simulink library "AMK_comms_plant_lib"  (R2022b)
settings: Solver=VariableStepAuto  StartTime=0.0  StopTime=10.0  RelTol=1e-3
libraries: dspstat3 x4, simulink x2
settings Model: Creator=LinF  LastModifiedBy=LinF

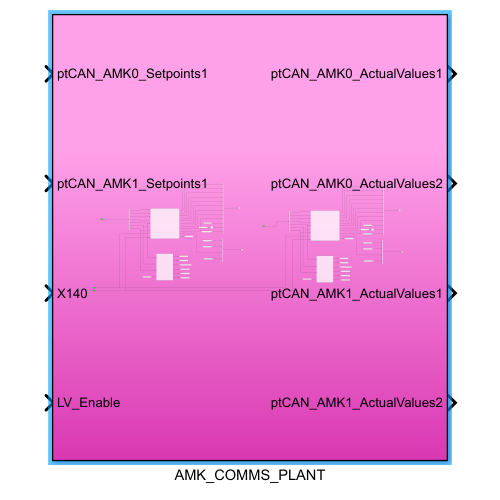
[thumbnail: Simulink's stored preview of the top-level diagram]
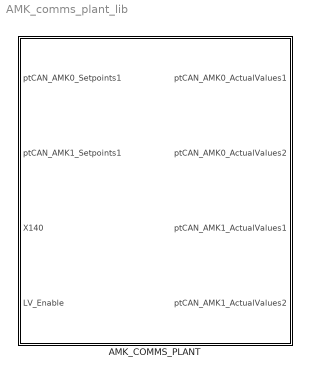
== system AMK_comms_plant_lib ==
  AMK_COMMS_PLANT : Subsystem

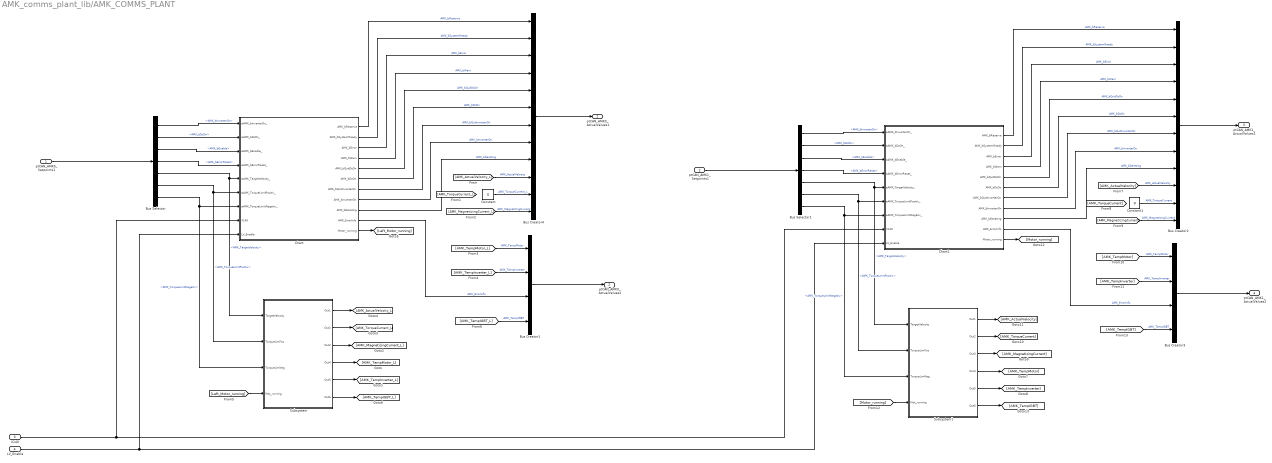
== system AMK_comms_plant_lib/AMK_COMMS_PLANT ==
  ptCAN_AMK0_Setpoints1 : Inport
  ptCAN_AMK1_Setpoints1 : Inport  Port=2
  X140 : Inport  Port=3
  LV_Enable : Inport  Port=4
  Bus Creator1 : BusCreator  Inputs=4
  Bus Creator2 : BusCreator  Inputs=12
  Bus Creator3 : BusCreator  Inputs=4
  Bus Creator4 : BusCreator  Inputs=12
  Bus Selector : BusSelector  OutputSignals=AMK_bInverterOn,AMK_bDcOn,AMK_bEnable,AMK_bErrorReset,AMK_TargetVelocity,AMK_TorqueLimitPositiv,AMK_TorqueLimitNegativ
  Bus Selector1 : BusSelector  OutputSignals=AMK_bInverterOn,AMK_bDcOn,AMK_bEnable,AMK_bErrorReset,AMK_TargetVelocity,AMK_TorqueLimitPositiv,AMK_TorqueLimitNegativ
  Chart : Stateflow chart  TreatAsAtomicUnit=on
  Chart1 : Stateflow chart  TreatAsAtomicUnit=on
  Constant : Constant  Value=0
  Constant1 : Constant  Value=0
  Subsystem : Subsystem
  Subsystem1 : Subsystem
  ptCAN_AMK0_ActualValues1 : Outport
  ptCAN_AMK0_ActualValues2 : Outport  Port=2
  ptCAN_AMK1_ActualValues1 : Outport  Port=3
  ptCAN_AMK1_ActualValues2 : Outport  Port=4
  wires:
  Subsystem/6(Out6) -> [AMK_TempIGBT_L]
  Subsystem/1(Out1) -> [AMK_ActualVelocity_L]
  Subsystem/2(Out2) -> [AMK_TorqueCurrent_L]
  Subsystem/3(Out3) -> [AMK_MagnetizingCurrent_L]
  Subsystem/4(Out4) -> [AMK_TempMotor_L]
  Subsystem/5(Out5) -> [AMK_TempInverter_L]
  [Left_Motor_running] -> Subsystem/4(Mot_running)
  Chart/11(Motor_running) -> [Left_Motor_running]
  Bus Selector/7 -> Subsystem/3(TorqueLimNeg), Chart/7(aAMK_TorqueLimitNegativ_)  "<AMK_TorqueLimitNegativ>"
  Bus Selector/6 -> Subsystem/2(TorqueLimPos), Chart/6(aAMK_TorqueLimitPositiv_)  "<AMK_TorqueLimitPositiv>"
  Bus Selector/5 -> Subsystem/1(TargetVelocity), Chart/5(aAMK_TargetVelocity_)  "<AMK_TargetVelocity>"
  Bus Selector/4 -> Chart/4(aAMK_bErrorReset_)  "<AMK_bErrorReset>"
  Bus Selector/3 -> Chart/3(aAMK_bEnable_)  "<AMK_bEnable>"
  Bus Selector/2 -> Chart/2(aAMK_bDcOn_)  "<AMK_bDcOn>"
  Bus Selector/1 -> Chart/1(aAMK_bInverterOn_)  "<AMK_bInverterOn>"
  ptCAN_AMK0_Setpoints1/1 -> Bus Selector/1
  Bus Creator1/1 -> ptCAN_AMK0_ActualValues2/1
  [AMK_TempMotor_L] -> Bus Creator1/1  "AMK_TempMotor"
  [AMK_TempIGBT_L] -> Bus Creator1/4  "AMK_TempIGBT"
  [AMK_TempInverter_L] -> Bus Creator1/2  "AMK_TempInverter"
  Chart/10(AMK_ErrorInfo) -> Bus Creator1/3  "AMK_ErrorInfo"
  LV_Enable/1 -> Chart1/9(LV_Enable), Chart/9(LV_Enable)
  Chart1/7(AMK_bQuitInverterOn) -> Bus Creator2/7  "AMK_bQuitInverterOn"
  [Motor_running] -> Subsystem1/4(Mot_running)
  X140/1 -> Chart/8(X140), Chart1/8(X140)
  Chart1/4(AMK_bWarn) -> Bus Creator2/4  "AMK_bWarn"
  Bus Creator2/1 -> ptCAN_AMK1_ActualValues1/1
  Chart1/10(AMK_ErrorInfo) -> Bus Creator3/3  "AMK_ErrorInfo"
  Chart1/6(AMK_bDcOn) -> Bus Creator2/6  "AMK_bDcOn"
  Chart1/1(AMK_bReserve) -> Bus Creator2/1  "AMK_bReserve"
  [AMK_TempInverter] -> Bus Creator3/2  "AMK_TempInverter"
  Bus Selector1/7 -> Subsystem1/3(TorqueLimNeg), Chart1/7(aAMK_TorqueLimitNegativ_)  "<AMK_TorqueLimitNegativ>"
  Chart1/3(AMK_bError) -> Bus Creator2/3  "AMK_bError"
  Chart1/9(AMK_bDerating) -> Bus Creator2/9  "AMK_bDerating"
  ptCAN_AMK1_Setpoints1/1 -> Bus Selector1/1
  Bus Selector1/4 -> Chart1/4(aAMK_bErrorReset_)  "<AMK_bErrorReset>"
  Bus Selector1/2 -> Chart1/2(aAMK_bDcOn_)  "<AMK_bDcOn>"
  [AMK_TempIGBT] -> Bus Creator3/4  "AMK_TempIGBT"
  Chart1/5(AMK_bQuitDcOn) -> Bus Creator2/5  "AMK_bQuitDcOn"
  Bus Selector1/1 -> Chart1/1(aAMK_bInverterOn_)  "<AMK_bInverterOn>"
  Subsystem1/3(Out3) -> [AMK_MagnetizingCurrent]
  Chart1/2(AMK_bSystemReady) -> Bus Creator2/2  "AMK_bSystemReady"
  Bus Selector1/5 -> Subsystem1/1(TargetVelocity), Chart1/5(aAMK_TargetVelocity_)  "<AMK_TargetVelocity>"
  [AMK_TempMotor] -> Bus Creator3/1  "AMK_TempMotor"
  Subsystem1/1(Out1) -> [AMK_ActualVelocity]
  Chart1/8(AMK_bInverterOn) -> Bus Creator2/8  "AMK_bInverterOn"
  Subsystem1/2(Out2) -> [AMK_TorqueCurrent]
  Subsystem1/6(Out6) -> [AMK_TempIGBT]
  Bus Selector1/3 -> Chart1/3(aAMK_bEnable_)  "<AMK_bEnable>"
  Subsystem1/5(Out5) -> [AMK_TempInverter]
  Chart1/11(Motor_running) -> [Motor_running]
  [AMK_ActualVelocity] -> Bus Creator2/10  "AMK_ActualVelocity"
  Subsystem1/4(Out4) -> [AMK_TempMotor]
  Bus Selector1/6 -> Subsystem1/2(TorqueLimPos), Chart1/6(aAMK_TorqueLimitPositiv_)  "<AMK_TorqueLimitPositiv>"
  Bus Creator3/1 -> ptCAN_AMK1_ActualValues2/1
  [AMK_MagnetizingCurrent] -> Bus Creator2/12  "AMK_MagnetizingCurrent"
  Chart/7(AMK_bQuitInverterOn) -> Bus Creator4/7  "AMK_bQuitInverterOn"
  [AMK_ActualVelocity_L] -> Bus Creator4/10  "AMK_ActualVelocity"
  Chart/8(AMK_bInverterOn) -> Bus Creator4/8  "AMK_bInverterOn"
  Chart/5(AMK_bQuitDcOn) -> Bus Creator4/5  "AMK_bQuitDcOn"
  Chart/2(AMK_bSystemReady) -> Bus Creator4/2  "AMK_bSystemReady"
  Chart/4(AMK_bWarn) -> Bus Creator4/4  "AMK_bWarn"
  Chart/9(AMK_bDerating) -> Bus Creator4/9  "AMK_bDerating"
  Chart/6(AMK_bDcOn) -> Bus Creator4/6  "AMK_bDcOn"
  Chart/3(AMK_bError) -> Bus Creator4/3  "AMK_bError"
  Bus Creator4/1 -> ptCAN_AMK0_ActualValues1/1
  [AMK_MagnetizingCurrent_L] -> Bus Creator4/12  "AMK_MagnetizingCurrent"
  Chart/1(AMK_bReserve) -> Bus Creator4/1  "AMK_bReserve"
  Constant/1 -> Bus Creator4/11  "AMK_TorqueCurrent_L"
  Constant1/1 -> Bus Creator2/11  "AMK_TorqueCurrent"

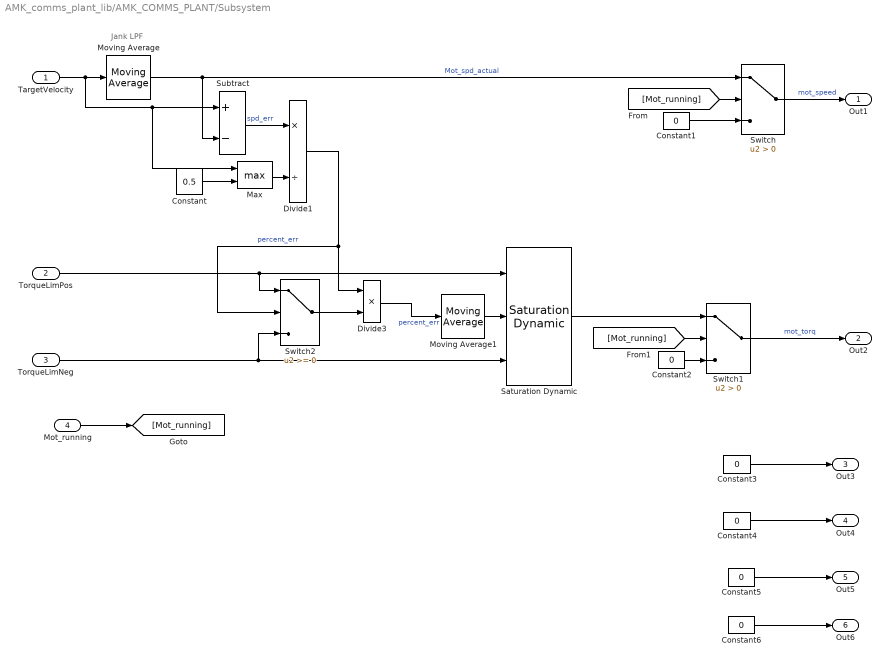
== system AMK_comms_plant_lib/AMK_COMMS_PLANT/Subsystem ==
  note: Jank LPF
  TargetVelocity : Inport
  TorqueLimPos : Inport  Port=2
  TorqueLimNeg : Inport  Port=3
  Mot_running : Inport  Port=4
  Constant : Constant  Value=0.5
  Constant1 : Constant  Value=0
  Constant2 : Constant  Value=0
  Constant{3..6} (4 alike) : Constant  Value=0  OutDataTypeStr=single
  Divide1 : Product  Inputs=*/
  Divide3 : Product  Inputs=**
  Max : MinMax  Function=max  Inputs=2
  Moving Average : dspstat3/Moving Average  Method=Sliding window  ForgettingFactorPort=off  SpecifyWindowLength=on  WindowLength=10  OverlapLength=9  AllowArbitraryInputLength=off  ForgettingFactor=0.9  SimulateUsing=Code generation
  Moving Average1 : dspstat3/Moving Average  Method=Sliding window  ForgettingFactorPort=off  SpecifyWindowLength=on  WindowLength=3  OverlapLength=2  AllowArbitraryInputLength=off  ForgettingFactor=0.9  SimulateUsing=Code generation
  Saturation Dynamic : simulink/Discontinuities/Saturation Dynamic  OutMin=[]  OutMax=[]  OutDataTypeStr=Inherit: Same as second input  OutDataType=fixdt(1, 16)  OutScaling=2^-10  DoSatur=off
  Subtract : Sum  Inputs=+-
  Switch : Switch  Criteria=u2 > Threshold  OutDataTypeStr=single  SaturateOnIntegerOverflow=off  InputSameDT=off
  Switch1 : Switch  Criteria=u2 > Threshold  OutDataTypeStr=single  SaturateOnIntegerOverflow=off  InputSameDT=off
  Switch2 : Switch  SaturateOnIntegerOverflow=off  InputSameDT=off
  Out1 : Outport
  Out2 : Outport  Port=2
  Out3 : Outport  Port=3
  Out4 : Outport  Port=4
  Out5 : Outport  Port=5
  Out6 : Outport  Port=6
  wires:
  Max/1 -> Divide1/2
  Constant/1 -> Max/2
  Constant6/1 -> Out6/1
  Divide3/1 -> Moving Average1/1  "percent_err"
  Moving Average1/1 -> Saturation Dynamic/2
  TorqueLimNeg/1 -> Saturation Dynamic/3, Switch2/3
  Switch2/1 -> Divide3/2
  TorqueLimPos/1 -> Switch2/1, Saturation Dynamic/1
  Constant5/1 -> Out5/1
  Constant4/1 -> Out4/1
  Constant3/1 -> Out3/1
  Divide1/1 -> Switch2/2, Divide3/1  "percent_err"
  TargetVelocity/1 -> Moving Average/1, Subtract/1, Max/1
  Subtract/1 -> Divide1/1  "spd_err"
  Switch1/1 -> Out2/1  "mot_torq"
  Saturation Dynamic/1 -> Switch1/1
  [Mot_running] -> Switch1/2
  Constant2/1 -> Switch1/3
  Moving Average/1 -> Subtract/2, Switch/1  "Mot_spd_actual"
  Constant1/1 -> Switch/3
  Switch/1 -> Out1/1  "mot_speed"
  [Mot_running] -> Switch/2
  Mot_running/1 -> [Mot_running]

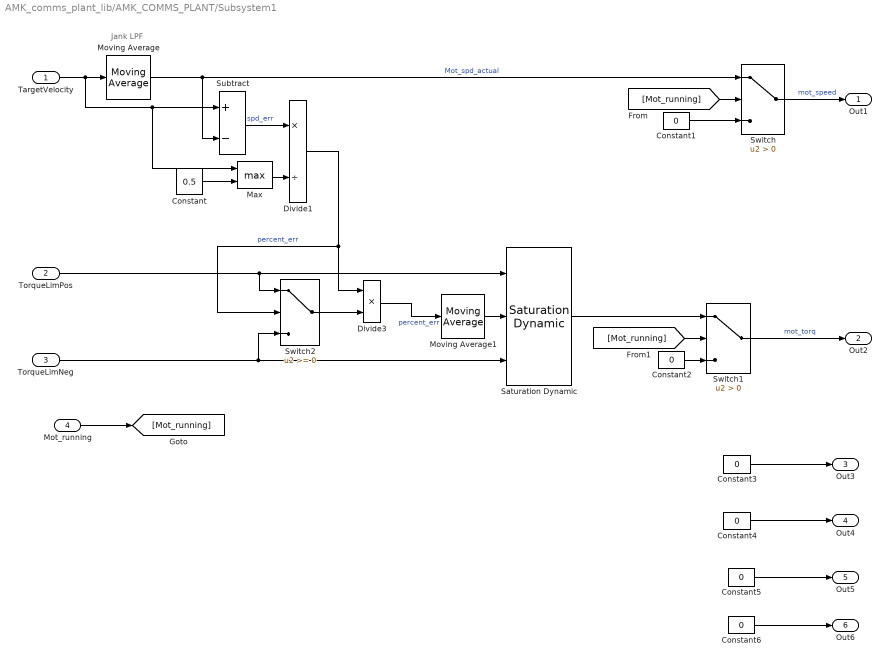
== system AMK_comms_plant_lib/AMK_COMMS_PLANT/Subsystem1 ==
  note: Jank LPF
  TargetVelocity : Inport
  TorqueLimPos : Inport  Port=2
  TorqueLimNeg : Inport  Port=3
  Mot_running : Inport  Port=4
  Constant : Constant  Value=0.5
  Constant1 : Constant  Value=0
  Constant2 : Constant  Value=0
  Constant{3..6} (4 alike) : Constant  Value=0  OutDataTypeStr=single
  Divide1 : Product  Inputs=*/
  Divide3 : Product  Inputs=**
  Max : MinMax  Function=max  Inputs=2
  Moving Average : dspstat3/Moving Average  Method=Sliding window  ForgettingFactorPort=off  SpecifyWindowLength=on  WindowLength=10  OverlapLength=9  AllowArbitraryInputLength=off  ForgettingFactor=0.9  SimulateUsing=Code generation
  Moving Average1 : dspstat3/Moving Average  Method=Sliding window  ForgettingFactorPort=off  SpecifyWindowLength=on  WindowLength=3  OverlapLength=2  AllowArbitraryInputLength=off  ForgettingFactor=0.9  SimulateUsing=Code generation
  Saturation Dynamic : simulink/Discontinuities/Saturation Dynamic  OutMin=[]  OutMax=[]  OutDataTypeStr=Inherit: Same as second input  OutDataType=fixdt(1, 16)  OutScaling=2^-10  DoSatur=off
  Subtract : Sum  Inputs=+-
  Switch : Switch  Criteria=u2 > Threshold  OutDataTypeStr=single  SaturateOnIntegerOverflow=off  InputSameDT=off
  Switch1 : Switch  Criteria=u2 > Threshold  OutDataTypeStr=single  SaturateOnIntegerOverflow=off  InputSameDT=off
  Switch2 : Switch  SaturateOnIntegerOverflow=off  InputSameDT=off
  Out1 : Outport
  Out2 : Outport  Port=2
  Out3 : Outport  Port=3
  Out4 : Outport  Port=4
  Out5 : Outport  Port=5
  Out6 : Outport  Port=6
  wires:
  Max/1 -> Divide1/2
  Constant/1 -> Max/2
  Constant6/1 -> Out6/1
  Divide3/1 -> Moving Average1/1  "percent_err"
  Moving Average1/1 -> Saturation Dynamic/2
  TorqueLimNeg/1 -> Saturation Dynamic/3, Switch2/3
  Switch2/1 -> Divide3/2
  TorqueLimPos/1 -> Switch2/1, Saturation Dynamic/1
  Constant5/1 -> Out5/1
  Constant4/1 -> Out4/1
  Constant3/1 -> Out3/1
  Divide1/1 -> Switch2/2, Divide3/1  "percent_err"
  TargetVelocity/1 -> Moving Average/1, Subtract/1, Max/1
  Subtract/1 -> Divide1/1  "spd_err"
  Switch1/1 -> Out2/1  "mot_torq"
  Saturation Dynamic/1 -> Switch1/1
  [Mot_running] -> Switch1/2
  Constant2/1 -> Switch1/3
  Moving Average/1 -> Subtract/2, Switch/1  "Mot_spd_actual"
  Constant1/1 -> Switch/3
  Switch/1 -> Out1/1  "mot_speed"
  [Mot_running] -> Switch/2
  Mot_running/1 -> [Mot_running]

== stateflow chart AMK_comms_plant_lib/AMK_COMMS_PLANT/Chart1 ==
  state AMK_idle
    en:
    AMK_bReserve = 0;
    AMK_bSystemReady = 0;
    AMK_bError = 0;
    AMK_bWarn = 0;
    AMK_bQuitDcOn = 0;
    AMK_bDcOn = 0;
    AMK_bQuitInverterOn = 0;
    AMK_bInverterOn = 0;
    AMK_bDerating = 0;
    AMK_ErrorInfo = 0;
    Motor_running = false;
  state LV_ON
    state Enable_System_Ready
      en:
      AMK_bSystemReady = 1;
    state bQuitDcOff
      en:
      AMK_bQuitDcOn = 0
    state Enable_Quit_Dc_On
      en:
      AMK_bQuitDcOn = 1;
      AMK_bDcOn = 1;
    state bDcOff
      en:
      AMK_bDcOn = 0
    state Inverter_Stuff2
      % (*3) and %(*4)
    state Inverter
    state bEnable_off
      en:
      AMK_bQuitDcOn = 0
    state Inventer_On
      en:
      AMK_bInverterOn = 1;
    state bInverter_off
      en:
      AMK_bInverterOn = 0
    state Quit_Inventer_On
      en:
      AMK_bQuitInverterOn =1;
    state Motor_running
      en:
      Motor_running = true;
    state Shut_off_start
      en:
      AMK_bQuitInverterOn =0;
    (default) -> Enable_System_Ready
    Enable_System_Ready -> (junction 99) : [aAMK_bDcOn_ == 1]
    (junction 99) -> Enable_Quit_Dc_On : after(250,msec)
    bDcOff -> bQuitDcOff
    Enable_Quit_Dc_On -> Inverter : [(abs(aAMK_TargetVelocity_) == 0) && ...
        | (abs(aAMK_TorqueLimitPositiv_) == 0) && ...
        | (abs(aAMK_TorqueLimitNegativ_) == 0)]
    Inverter_Stuff2 -> bDcOff : [aAMK_bDcOn_ == 0]
    bEnable_off -> Inverter_Stuff2
    Inverter -> (junction 101) : [(aAMK_bEnable_ == 1) && ...
        | (aAMK_bInverterOn_ == 1)]
    (junction 101) -> Inventer_On : after(250,msec)
    bInverter_off -> bEnable_off : [aAMK_bEnable_ == 0]
    Inventer_On -> Quit_Inventer_On : [X140 == 1]
    Shut_off_start -> bInverter_off [order 2] : [aAMK_bInverterOn_ == 0]
    Shut_off_start -> Quit_Inventer_On [order 1] : [X140 == 1]
    Quit_Inventer_On -> Motor_running : after(250,msec)
    Motor_running -> Shut_off_start : [X140 == 0]
  (default) -> AMK_idle
  AMK_idle -> LV_ON : [LV_Enable == 1]
  LV_ON -> AMK_idle : [LV_Enable == 0]
  data: aAMK_bInverterOn_ input; aAMK_bDcOn_ input; aAMK_bEnable_ input; aAMK_bErrorReset_ input; aAMK_TargetVelocity_ input; aAMK_TorqueLimitPositiv_ input; aAMK_TorqueLimitNegativ_ input; AMK_bReserve output uint8; AMK_bSystemReady output uint8; AMK_bError output uint8; AMK_bWarn output uint8; AMK_bQuitDcOn output uint8; AMK_bDcOn output uint8; AMK_bQuitInverterOn output uint8; AMK_bInverterOn output uint8; AMK_bDerating output uint8; AMK_ErrorInfo output int32; Motor_running output boolean =false; X140 input; LV_Enable input

== stateflow chart AMK_comms_plant_lib/AMK_COMMS_PLANT/Chart ==
  state AMK_idle
    en:
    AMK_bReserve = 0;
    AMK_bSystemReady = 0;
    AMK_bError = 0;
    AMK_bWarn = 0;
    AMK_bQuitDcOn = 0;
    AMK_bDcOn = 0;
    AMK_bQuitInverterOn = 0;
    AMK_bInverterOn = 0;
    AMK_bDerating = 0;
    AMK_ErrorInfo = 0;
    Motor_running = false;
  state LV_ON
    state Enable_System_Ready
      en:
      AMK_bSystemReady = 1;
    state bQuitDcOff
      en:
      AMK_bQuitDcOn = 0
    state Enable_Quit_Dc_On
      en:
      AMK_bQuitDcOn = 1;
      AMK_bDcOn = 1;
    state bDcOff
      en:
      AMK_bDcOn = 0
    state Inverter_Stuff2
      % (*3) and %(*4)
    state Inverter
    state bEnable_off
      en:
      AMK_bQuitDcOn = 0
    state Inventer_On
      en:
      AMK_bInverterOn = 1;
    state bInverter_off
      en:
      AMK_bInverterOn = 0
    state Quit_Inventer_On
      en:
      AMK_bQuitInverterOn =1;
    state Motor_running
      en:
      Motor_running = true;
    state Shut_off_start
      en:
      AMK_bQuitInverterOn =0;
    (default) -> Enable_System_Ready
    Enable_System_Ready -> (junction 99) : [aAMK_bDcOn_ == 1]
    (junction 99) -> Enable_Quit_Dc_On : after(250,msec)
    bDcOff -> bQuitDcOff
    Enable_Quit_Dc_On -> Inverter : [(abs(aAMK_TargetVelocity_) == 0) && ...
        | (abs(aAMK_TorqueLimitPositiv_) == 0) && ...
        | (abs(aAMK_TorqueLimitNegativ_) == 0)]
    Inverter_Stuff2 -> bDcOff : [aAMK_bDcOn_ == 0]
    bEnable_off -> Inverter_Stuff2
    Inverter -> (junction 101) : [(aAMK_bEnable_ == 1) && ...
        | (aAMK_bInverterOn_ == 1)]
    (junction 101) -> Inventer_On : after(250,msec)
    bInverter_off -> bEnable_off : [aAMK_bEnable_ == 0]
    Inventer_On -> Quit_Inventer_On : [X140 == 1]
    Shut_off_start -> bInverter_off [order 2] : [aAMK_bInverterOn_ == 0]
    Shut_off_start -> Quit_Inventer_On [order 1] : [X140 == 1]
    Quit_Inventer_On -> Motor_running : after(250,msec)
    Motor_running -> Shut_off_start : [X140 == 0]
  (default) -> AMK_idle
  AMK_idle -> LV_ON : [LV_Enable == 1]
  LV_ON -> AMK_idle : [LV_Enable == 0]
  data: aAMK_bInverterOn_ input; aAMK_bDcOn_ input; aAMK_bEnable_ input; aAMK_bErrorReset_ input; aAMK_TargetVelocity_ input; aAMK_TorqueLimitPositiv_ input; aAMK_TorqueLimitNegativ_ input; AMK_bReserve output uint8; AMK_bSystemReady output uint8; AMK_bError output uint8; AMK_bWarn output uint8; AMK_bQuitDcOn output uint8; AMK_bDcOn output uint8; AMK_bQuitInverterOn output uint8; AMK_bInverterOn output uint8; AMK_bDerating output uint8; AMK_ErrorInfo output int32; Motor_running output boolean =false; X140 input; LV_Enable input
